simulink model "PI_Contoller"  (R2020b)
settings: Solver=VariableStepAuto  StartTime=0.0  StopTime=10.0  RelTol=1e-3
values from neighbouring files (symbols this model uses):
  Ki = 40.0    [Cruise_DataDictionary.sldd]
  Kp = 800.0    [Cruise_DataDictionary.sldd]
settings Model: DataDictionary=Cruise_DataDictionary.sldd  Creator=Sourav Kumar  LastModifiedBy=Sourav Kumar
settings DataIOCC: SaveOutput=off  SaveTime=off

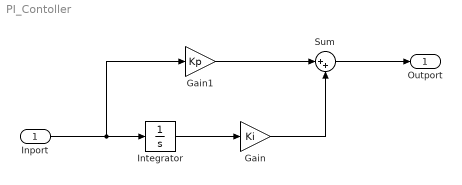
== system PI_Contoller ==
  Inport : Inport  OutDataTypeStr=double  PortDimensions=1  SampleTime=0
  Gain : Gain  Gain=Ki
  Gain1 : Gain  Gain=Kp
  Integrator : Integrator
  Sum : Sum  Inputs=|++
  Outport : Outport  OutDataTypeStr=double  PortDimensions=1  SampleTime=0
  wires:
  Gain/1 -> Sum/2
  Inport/1 -> Integrator/1, Gain1/1
  Integrator/1 -> Gain/1
  Sum/1 -> Outport/1
  Gain1/1 -> Sum/1
